simulink subsystem "HI_FastAnalogInputs"  (R2019b)
settings: Solver=VariableStepAuto  StartTime=0.0  StopTime=10.0  RelTol=1e-3
libraries: c2802xlib x4
settings Model: Creator=Nick  LastModifiedBy=zacha

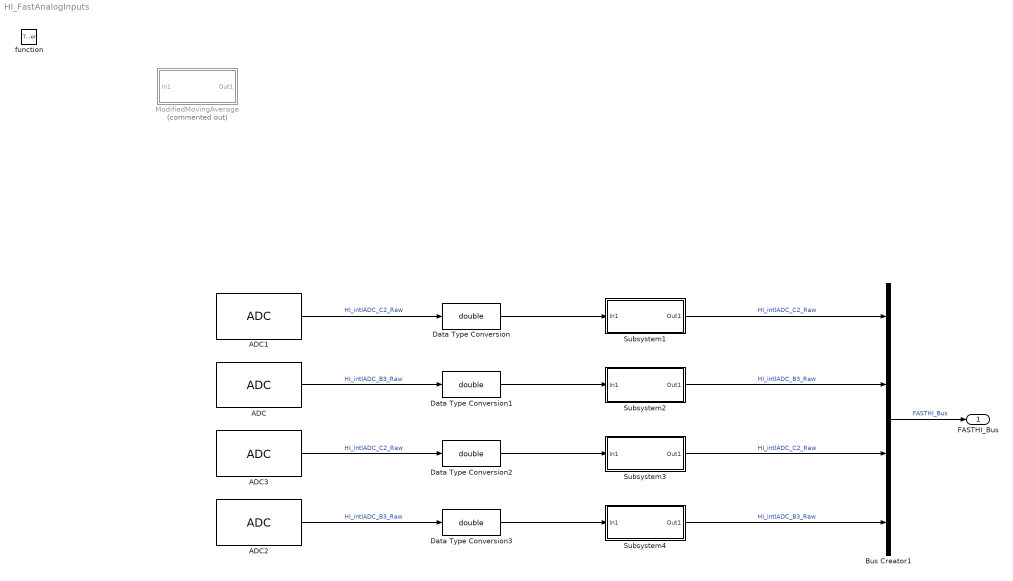
== system HI_FastAnalogInputs ==
  function : TriggerPort  TriggerType=function-call  VariantControl=Variant
  ADC : c2802xlib/ADC  blkParamProc=C2000_Type4  ADCModule=B  samplingMode=Single sample mode  ADCResolution=12-bit (Single-ended input)  useSOC1=SOC3  useSOC2=SOC0_SOC1  SOCAcquisitionWindow=15  SOCTriggerSource=Software  SOCInterruptTrigger=No ADCINT  Ts=-1  dType=uint16  postInterrupt=off  interruptSel=ADCINT1  ADCINTContinuous=on  endma=off  chdma=1  conv1=ADCINA0  conv2=ADCINA0 and ADCINB0  conv1_Type4=ADCIN3  conv2_Type4=ADCIN2 and ADCIN3
      settings: SourceProductName=Embedded Coder Support Package for Texas Instruments C2000 Processors
  ADC1 : c2802xlib/ADC  blkParamProc=C2000_Type4  ADCModule=C  samplingMode=Single sample mode  ADCResolution=12-bit (Single-ended input)  useSOC1=SOC3  useSOC2=SOC0_SOC1  SOCAcquisitionWindow=15  SOCTriggerSource=Software  SOCInterruptTrigger=No ADCINT  Ts=-1  dType=uint16  postInterrupt=off  interruptSel=ADCINT1  ADCINTContinuous=on  endma=off  chdma=1  conv1=ADCINA0  conv2=ADCINA0 and ADCINB0  conv1_Type4=ADCIN3  conv2_Type4=ADCIN2 and ADCIN3
      settings: SourceProductName=Embedded Coder Support Package for Texas Instruments C2000 Processors
  ADC2 : c2802xlib/ADC  blkParamProc=C2000_Type4  ADCModule=B  samplingMode=Single sample mode  ADCResolution=12-bit (Single-ended input)  useSOC1=SOC2  useSOC2=SOC0_SOC1  SOCAcquisitionWindow=15  SOCTriggerSource=Software  SOCInterruptTrigger=No ADCINT  Ts=-1  dType=uint16  postInterrupt=off  interruptSel=ADCINT1  ADCINTContinuous=on  endma=off  chdma=1  conv1=ADCINA0  conv2=ADCINA0 and ADCINB0  conv1_Type4=ADCIN2  conv2_Type4=ADCIN2 and ADCIN3
      settings: SourceProductName=Embedded Coder Support Package for Texas Instruments C2000 Processors
  ADC3 : c2802xlib/ADC  blkParamProc=C2000_Type4  ADCModule=C  samplingMode=Single sample mode  ADCResolution=12-bit (Single-ended input)  useSOC1=SOC2  useSOC2=SOC0_SOC1  SOCAcquisitionWindow=15  SOCTriggerSource=Software  SOCInterruptTrigger=No ADCINT  Ts=-1  dType=uint16  postInterrupt=off  interruptSel=ADCINT1  ADCINTContinuous=on  endma=off  chdma=1  conv1=ADCINA0  conv2=ADCINA0 and ADCINB0  conv1_Type4=ADCIN2  conv2_Type4=ADCIN2 and ADCIN3
      settings: SourceProductName=Embedded Coder Support Package for Texas Instruments C2000 Processors
  Bus Creator1 : BusCreator  Inputs=4
  Data Type Conversion{,1..3} (4 alike) : DataTypeConversion  OutDataTypeStr=double
  ModifiedMovingAverage : Subsystem  Commented=on
  Subsystem1 : Subsystem
  Subsystem2 : Subsystem
  Subsystem3 : Subsystem
  Subsystem4 : Subsystem
  FASTHI_Bus : Outport
  wires:
  Subsystem1/1(Out1) -> Bus Creator1/1  "HI_intlADC_C2_Raw"
  ADC1/1 -> Data Type Conversion/1  "HI_intlADC_C2_Raw"
  Data Type Conversion1/1 -> Subsystem2/1(In1)
  Bus Creator1/1 -> FASTHI_Bus/1  "FASTHI_Bus"
  Data Type Conversion/1 -> Subsystem1/1(In1)
  Subsystem2/1(Out1) -> Bus Creator1/2  "HI_intlADC_B3_Raw"
  ADC/1 -> Data Type Conversion1/1  "HI_intlADC_B3_Raw"
  Subsystem4/1(Out1) -> Bus Creator1/4  "HI_intlADC_B3_Raw"
  Data Type Conversion3/1 -> Subsystem4/1(In1)
  ADC3/1 -> Data Type Conversion2/1  "HI_intlADC_C2_Raw"
  Data Type Conversion2/1 -> Subsystem3/1(In1)
  ADC2/1 -> Data Type Conversion3/1  "HI_intlADC_B3_Raw"
  Subsystem3/1(Out1) -> Bus Creator1/3  "HI_intlADC_C2_Raw"

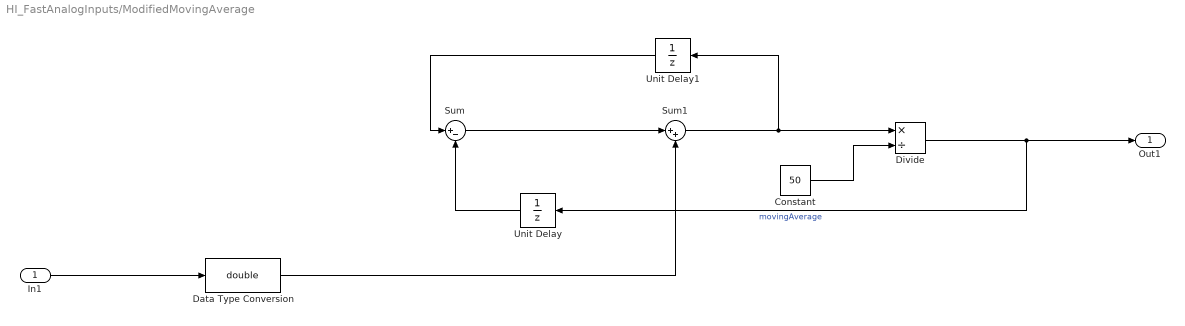
== system HI_FastAnalogInputs/ModifiedMovingAverage ==
  In1 : Inport
  Constant : Constant  Value=50
  Data Type Conversion : DataTypeConversion  OutDataTypeStr=double
  Divide : Product  Inputs=*/
  Sum : Sum  Inputs=|+-
  Sum1 : Sum  Inputs=|++
  Unit Delay : UnitDelay  SampleTime=-1  HasFrameUpgradeWarning=on
  Unit Delay1 : UnitDelay  SampleTime=-1  HasFrameUpgradeWarning=on
  Out1 : Outport
  wires:
  Unit Delay/1 -> Sum/2
  Unit Delay1/1 -> Sum/1
  Divide/1 -> Out1/1, Unit Delay/1  "movingAverage"
  Constant/1 -> Divide/2
  Sum1/1 -> Divide/1, Unit Delay1/1
  Sum/1 -> Sum1/1
  Data Type Conversion/1 -> Sum1/2
  In1/1 -> Data Type Conversion/1

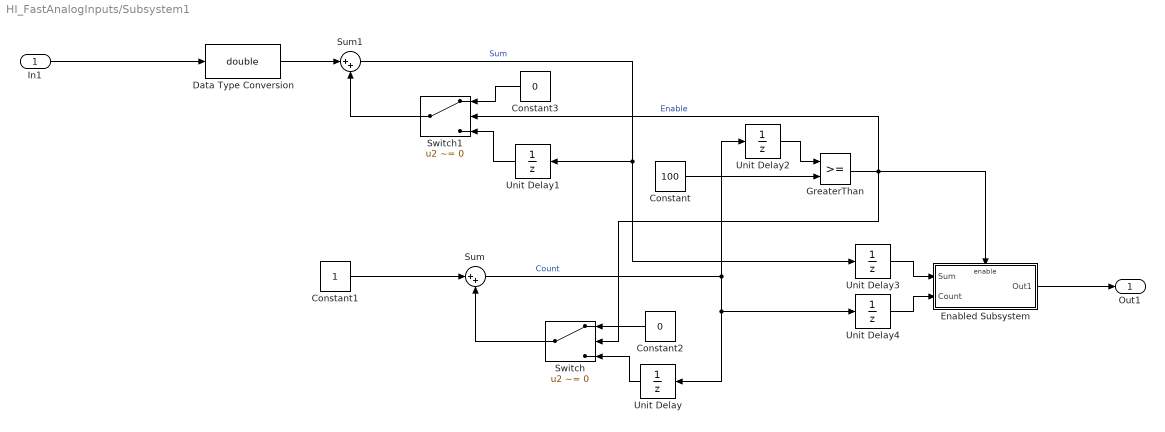
== system HI_FastAnalogInputs/Subsystem1 ==
  In1 : Inport
  Constant : Constant  Value=100
  Constant1 : Constant
  Constant2 : Constant  Value=0
  Constant3 : Constant  Value=0
  Data Type Conversion : DataTypeConversion  OutDataTypeStr=double
  Enabled Subsystem : Subsystem  TreatAsAtomicUnit=on
  GreaterThan : RelationalOperator  OutDataTypeStr=boolean  RndMeth=Simplest
  Sum : Sum  Inputs=|++
  Sum1 : Sum  Inputs=|++
  Switch : Switch  Criteria=u2 ~= 0  Threshold=50
  Switch1 : Switch  Criteria=u2 ~= 0  Threshold=50
  Unit Delay{,1..4} (5 alike) : UnitDelay  SampleTime=-1  HasFrameUpgradeWarning=on
  Out1 : Outport
  wires:
  Unit Delay3/1 -> Enabled Subsystem/1(Sum)
  Unit Delay4/1 -> Enabled Subsystem/2(Count)
  Unit Delay2/1 -> GreaterThan/1
  Switch1/1 -> Sum1/2
  Constant3/1 -> Switch1/1
  Unit Delay1/1 -> Switch1/3
  Data Type Conversion/1 -> Sum1/1
  Switch/1 -> Sum/2
  Constant2/1 -> Switch/1
  Unit Delay/1 -> Switch/3
  Constant1/1 -> Sum/1
  GreaterThan/1 -> Enabled Subsystem/Enable, Switch/2, Switch1/2  "Enable"
  Sum/1 -> Unit Delay2/1, Unit Delay/1, Unit Delay4/1  "Count"
  Sum1/1 -> Unit Delay1/1, Unit Delay3/1  "Sum"
  Constant/1 -> GreaterThan/2
  Enabled Subsystem/1(Out1) -> Out1/1
  In1/1 -> Data Type Conversion/1

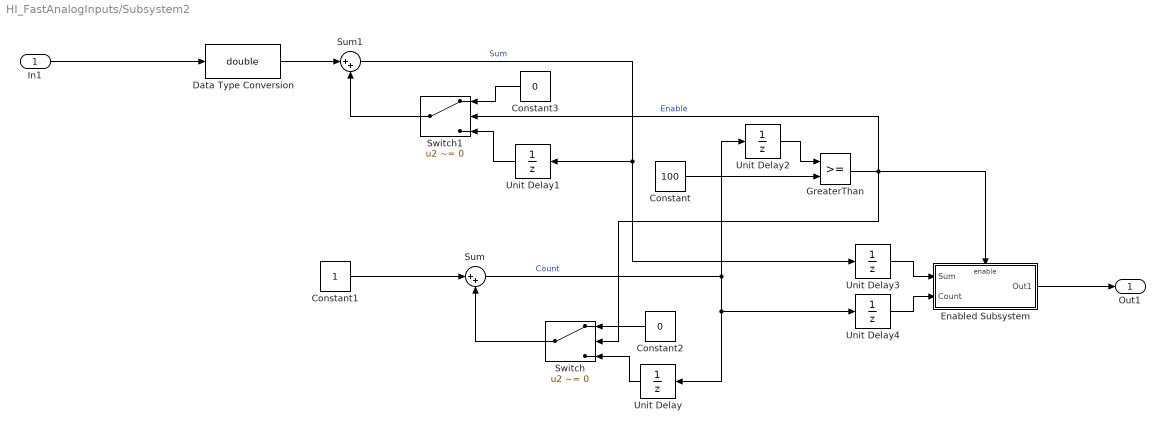
== system HI_FastAnalogInputs/Subsystem2 ==
  In1 : Inport
  Constant : Constant  Value=100
  Constant1 : Constant
  Constant2 : Constant  Value=0
  Constant3 : Constant  Value=0
  Data Type Conversion : DataTypeConversion  OutDataTypeStr=double
  Enabled Subsystem : Subsystem  TreatAsAtomicUnit=on
  GreaterThan : RelationalOperator  OutDataTypeStr=boolean  RndMeth=Simplest
  Sum : Sum  Inputs=|++
  Sum1 : Sum  Inputs=|++
  Switch : Switch  Criteria=u2 ~= 0  Threshold=50
  Switch1 : Switch  Criteria=u2 ~= 0  Threshold=50
  Unit Delay{,1..4} (5 alike) : UnitDelay  SampleTime=-1  HasFrameUpgradeWarning=on
  Out1 : Outport
  wires:
  Unit Delay3/1 -> Enabled Subsystem/1(Sum)
  Unit Delay4/1 -> Enabled Subsystem/2(Count)
  Unit Delay2/1 -> GreaterThan/1
  Switch1/1 -> Sum1/2
  Constant3/1 -> Switch1/1
  Unit Delay1/1 -> Switch1/3
  Data Type Conversion/1 -> Sum1/1
  Switch/1 -> Sum/2
  Constant2/1 -> Switch/1
  Unit Delay/1 -> Switch/3
  Constant1/1 -> Sum/1
  GreaterThan/1 -> Enabled Subsystem/Enable, Switch/2, Switch1/2  "Enable"
  Sum/1 -> Unit Delay2/1, Unit Delay/1, Unit Delay4/1  "Count"
  Sum1/1 -> Unit Delay1/1, Unit Delay3/1  "Sum"
  Constant/1 -> GreaterThan/2
  Enabled Subsystem/1(Out1) -> Out1/1
  In1/1 -> Data Type Conversion/1

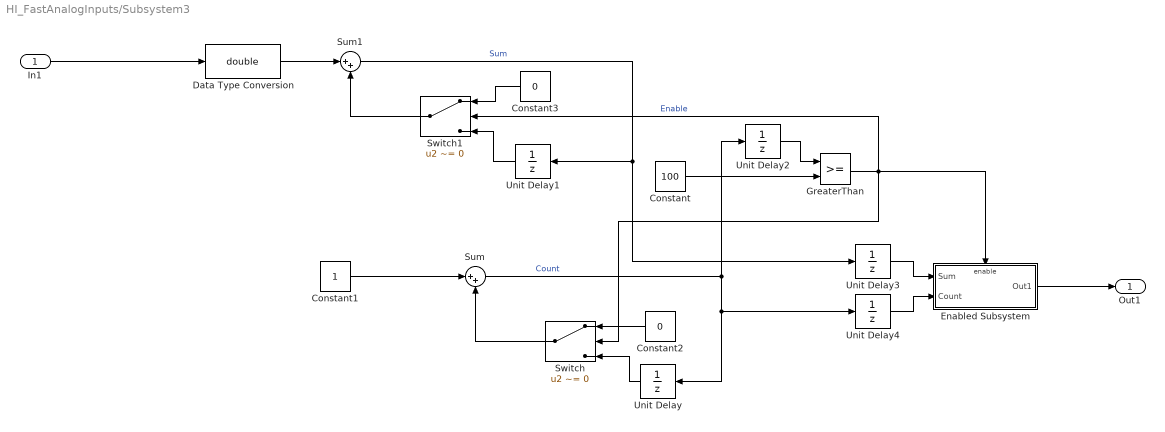
== system HI_FastAnalogInputs/Subsystem3 ==
  In1 : Inport
  Constant : Constant  Value=100
  Constant1 : Constant
  Constant2 : Constant  Value=0
  Constant3 : Constant  Value=0
  Data Type Conversion : DataTypeConversion  OutDataTypeStr=double
  Enabled Subsystem : Subsystem  TreatAsAtomicUnit=on
  GreaterThan : RelationalOperator  OutDataTypeStr=boolean  RndMeth=Simplest
  Sum : Sum  Inputs=|++
  Sum1 : Sum  Inputs=|++
  Switch : Switch  Criteria=u2 ~= 0  Threshold=50
  Switch1 : Switch  Criteria=u2 ~= 0  Threshold=50
  Unit Delay{,1..4} (5 alike) : UnitDelay  SampleTime=-1  HasFrameUpgradeWarning=on
  Out1 : Outport
  wires:
  Unit Delay3/1 -> Enabled Subsystem/1(Sum)
  Unit Delay4/1 -> Enabled Subsystem/2(Count)
  Unit Delay2/1 -> GreaterThan/1
  Switch1/1 -> Sum1/2
  Constant3/1 -> Switch1/1
  Unit Delay1/1 -> Switch1/3
  Data Type Conversion/1 -> Sum1/1
  Switch/1 -> Sum/2
  Constant2/1 -> Switch/1
  Unit Delay/1 -> Switch/3
  Constant1/1 -> Sum/1
  GreaterThan/1 -> Enabled Subsystem/Enable, Switch/2, Switch1/2  "Enable"
  Sum/1 -> Unit Delay2/1, Unit Delay/1, Unit Delay4/1  "Count"
  Sum1/1 -> Unit Delay1/1, Unit Delay3/1  "Sum"
  Constant/1 -> GreaterThan/2
  Enabled Subsystem/1(Out1) -> Out1/1
  In1/1 -> Data Type Conversion/1

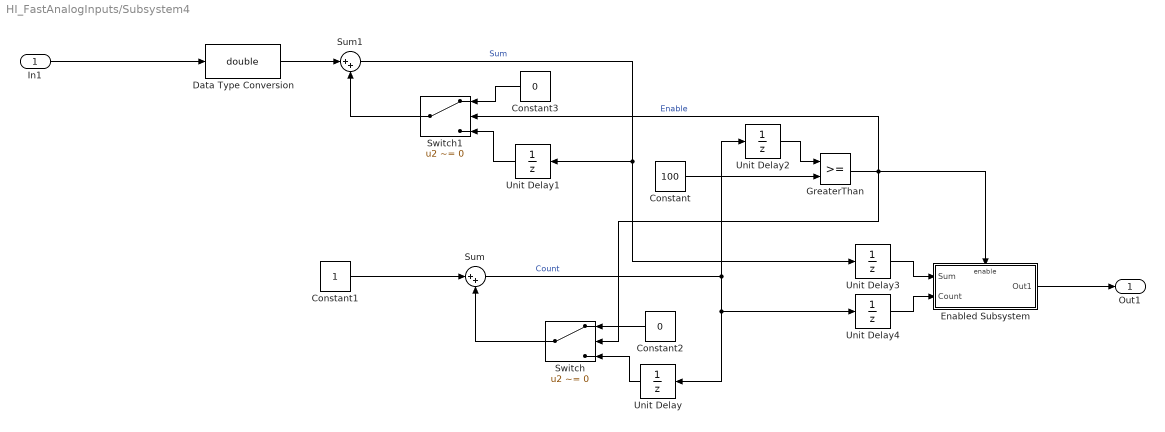
== system HI_FastAnalogInputs/Subsystem4 ==
  In1 : Inport
  Constant : Constant  Value=100
  Constant1 : Constant
  Constant2 : Constant  Value=0
  Constant3 : Constant  Value=0
  Data Type Conversion : DataTypeConversion  OutDataTypeStr=double
  Enabled Subsystem : Subsystem  TreatAsAtomicUnit=on
  GreaterThan : RelationalOperator  OutDataTypeStr=boolean  RndMeth=Simplest
  Sum : Sum  Inputs=|++
  Sum1 : Sum  Inputs=|++
  Switch : Switch  Criteria=u2 ~= 0  Threshold=50
  Switch1 : Switch  Criteria=u2 ~= 0  Threshold=50
  Unit Delay{,1..4} (5 alike) : UnitDelay  SampleTime=-1  HasFrameUpgradeWarning=on
  Out1 : Outport
  wires:
  Unit Delay3/1 -> Enabled Subsystem/1(Sum)
  Unit Delay4/1 -> Enabled Subsystem/2(Count)
  Unit Delay2/1 -> GreaterThan/1
  Switch1/1 -> Sum1/2
  Constant3/1 -> Switch1/1
  Unit Delay1/1 -> Switch1/3
  Data Type Conversion/1 -> Sum1/1
  Switch/1 -> Sum/2
  Constant2/1 -> Switch/1
  Unit Delay/1 -> Switch/3
  Constant1/1 -> Sum/1
  GreaterThan/1 -> Enabled Subsystem/Enable, Switch/2, Switch1/2  "Enable"
  Sum/1 -> Unit Delay2/1, Unit Delay/1, Unit Delay4/1  "Count"
  Sum1/1 -> Unit Delay1/1, Unit Delay3/1  "Sum"
  Constant/1 -> GreaterThan/2
  Enabled Subsystem/1(Out1) -> Out1/1
  In1/1 -> Data Type Conversion/1

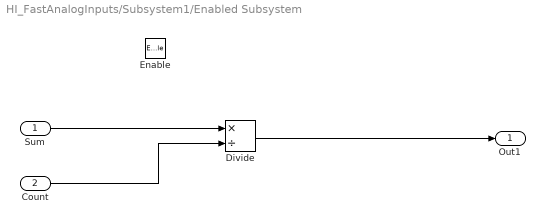
== system HI_FastAnalogInputs/Subsystem1/Enabled Subsystem ==
  Sum : Inport
  Count : Inport  Port=2
  Enable : EnablePort
  Divide : Product  Inputs=*/
  Out1 : Outport
  wires:
  Divide/1 -> Out1/1
  Count/1 -> Divide/2
  Sum/1 -> Divide/1

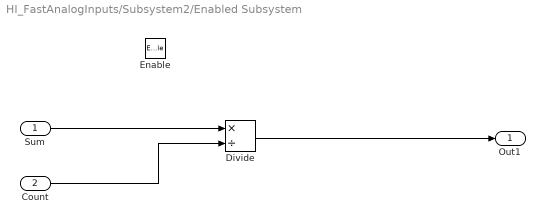
== system HI_FastAnalogInputs/Subsystem2/Enabled Subsystem ==
  Sum : Inport
  Count : Inport  Port=2
  Enable : EnablePort
  Divide : Product  Inputs=*/
  Out1 : Outport
  wires:
  Divide/1 -> Out1/1
  Count/1 -> Divide/2
  Sum/1 -> Divide/1

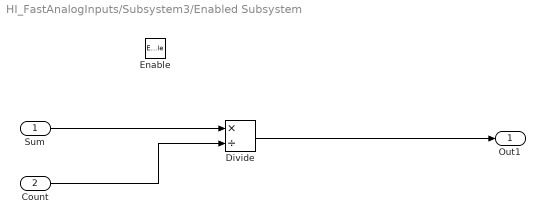
== system HI_FastAnalogInputs/Subsystem3/Enabled Subsystem ==
  Sum : Inport
  Count : Inport  Port=2
  Enable : EnablePort
  Divide : Product  Inputs=*/
  Out1 : Outport
  wires:
  Divide/1 -> Out1/1
  Count/1 -> Divide/2
  Sum/1 -> Divide/1

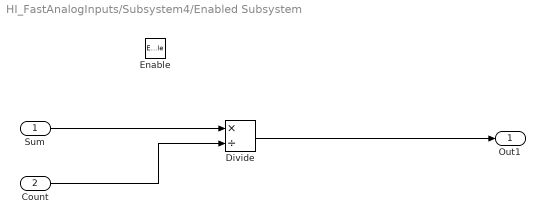
== system HI_FastAnalogInputs/Subsystem4/Enabled Subsystem ==
  Sum : Inport
  Count : Inport  Port=2
  Enable : EnablePort
  Divide : Product  Inputs=*/
  Out1 : Outport
  wires:
  Divide/1 -> Out1/1
  Count/1 -> Divide/2
  Sum/1 -> Divide/1
